simulink model "specification_1"  (Simulink 4.00)
settings: Solver=ode45  StartTime=0.0  StopTime=10.0  RelTol=1e-3
libraries: simulink3 x1
settings Model: LastModifiedBy=Administrator  Refine=5  BlockReductionOpt=off

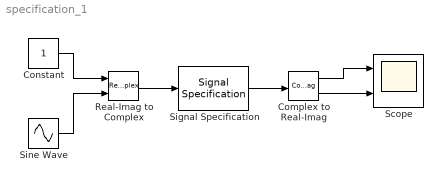
== system specification_1 ==
  Complex to Real-Imag : ComplexToRealImag  Output=RealAndImag
  Constant : Constant  Value=1
  Real-Imag to Complex : RealImagToComplex  Input=RealAndImag  ConstantPart=0
  Scope : Scope  NumInputPorts=2
      settings: TimeRange=auto  YMin=-5~-5  YMax=5~5  SaveToWorkspace=off  SaveName=ScopeData  LimitDataPoints=on  MaxDataPoints=5000
  Signal Specification : simulink3/Signals & Systems/Signal Specification  D=-1  Ts=-1  DataType=auto
      settings: SignalType=complex
  Sine Wave : Sin  Amplitude=1  Frequency=2*pi  Phase=0  SampleTime=0
  wires:
  Real-Imag to Complex/1 -> Signal Specification/1
  Constant/1 -> Real-Imag to Complex/1
  Sine Wave/1 -> Real-Imag to Complex/2
  Signal Specification/1 -> Complex to Real-Imag/1
  Complex to Real-Imag/1 -> Scope/1
  Complex to Real-Imag/2 -> Scope/2
